simulink model "SIMULACION_DEFINITIVA"  (R2019b)
settings: Solver=VariableStepAuto  StartTime=0.0  StopTime=10.0  RelTol=1e-3
values from neighbouring files (symbols this model uses):
  A = double(A)    [CODIGO_FINAL_PROYECTO.m]
  B = double(B)    [CODIGO_FINAL_PROYECTO.m]
  C = [1 0 0 0;0 0 1 0]    [CODIGO_FINAL_PROYECTO.m]
  K = lqr(A,B,Q,R)    [CODIGO_FINAL_PROYECTO.m]
  L = lqr(A',C',E*Sxi*E',Seta)'    [CODIGO_FINAL_PROYECTO.m]
  r = 0    [CODIGO_FINAL_PROYECTO.m]
  Seta = diag([0.01^2,0.01^2])    [CODIGO_FINAL_PROYECTO.m]
  Sxi = diag([0.05^2,0.05^2])    [CODIGO_FINAL_PROYECTO.m]
  UEQ = 0    [CODIGO_FINAL_PROYECTO.m]
  x0 = [179*pi/180;0;0*pi/180;0]    [CODIGO_FINAL_PROYECTO.m]
  XEQ = [pi;0;0;0]    [CODIGO_FINAL_PROYECTO.m]
  xh0 = [179*pi/180;0;0*pi/180;0]*1.05    [CODIGO_FINAL_PROYECTO.m]
  YEQ = [pi;0]    [CODIGO_FINAL_PROYECTO.m]
settings Model: Creator=Raffa  LastModifiedBy=Raffa

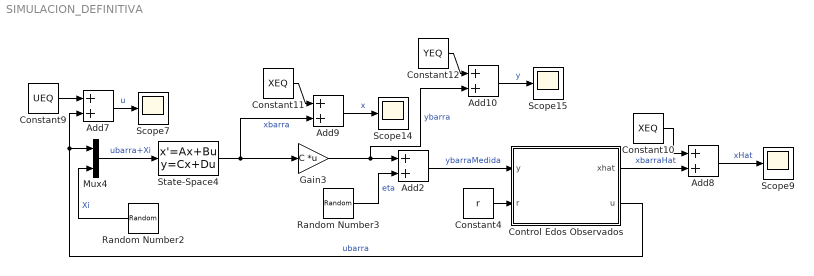
== system SIMULACION_DEFINITIVA ==
  Add{2,7..10} (5 alike) : Sum
  Constant10 : Constant  Value=XEQ
  Constant11 : Constant  Value=XEQ
  Constant12 : Constant  Value=YEQ
  Constant4 : Constant  Value=r  VectorParams1D=off
  Constant9 : Constant  Value=UEQ
  Control Edos Observados : Subsystem
  Gain3 : Gain  Gain=C  Multiplication=Matrix(K*u)
  Mux4 : Mux  Inputs=2
  Random Number2 : RandomNumber  Mean=[0;0]  Variance=[Sxi(1,1);Sxi(2,2)]  Seed=[1;2]  SampleTime=0.001  VectorParams1D=off
  Random Number3 : RandomNumber  Mean=[0;0]  Variance=[Seta(1,1);Seta(2,2)]  Seed=[3;4]  SampleTime=0.001  VectorParams1D=off
  Scope{7,9,14..15} (4 alike) : Scope
  State-Space4 : StateSpace  A=A  B=[B E]  C=eye(4)  D=zeros(4,3)  InitialCondition=x0-XEQ
  wires:
  Control Edos Observados/2(u) -> Add7/2, Mux4/1  "ubarra"
  Mux4/1 -> State-Space4/1  "ubarra+Xi"
  Gain3/1 -> Add10/2, Add2/1  "ybarra"
  Constant10/1 -> Add8/1
  Random Number2/1 -> Mux4/2  "Xi"
  Add8/1 -> Scope9/1  "xHat"
  Add10/1 -> Scope15/1  "y"
  Random Number3/1 -> Add2/2  "eta"
  Add7/1 -> Scope7/1  "u"
  Constant9/1 -> Add7/1
  Add2/1 -> Control Edos Observados/1(y)  "ybarraMedida"
  State-Space4/1 -> Gain3/1, Add9/2  "xbarra"
  Constant11/1 -> Add9/1
  Constant4/1 -> Control Edos Observados/2(r)
  Control Edos Observados/1(xhat) -> Add8/2  "xbarraHat"
  Add9/1 -> Scope14/1  "x"
  Constant12/1 -> Add10/1

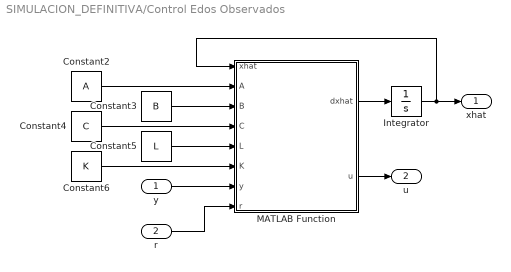
== system SIMULACION_DEFINITIVA/Control Edos Observados ==
  y : Inport
  r : Inport  Port=2
  Constant2 : Constant  Value=A  VectorParams1D=off
  Constant3 : Constant  Value=B  VectorParams1D=off
  Constant4 : Constant  Value=C  VectorParams1D=off
  Constant5 : Constant  Value=L  VectorParams1D=off
  Constant6 : Constant  Value=K  VectorParams1D=off
  Integrator : Integrator  InitialCondition=xh0-XEQ
  MATLAB Function : MATLAB Function  TreatAsAtomicUnit=on
  xhat : Outport
  u : Outport  Port=2
  wires:
  r/1 -> MATLAB Function/8(r)
  y/1 -> MATLAB Function/7(y)
  Constant4/1 -> MATLAB Function/4(C)
  Constant6/1 -> MATLAB Function/6(K)
  Constant5/1 -> MATLAB Function/5(L)
  Integrator/1 -> MATLAB Function/1(xhat), xhat/1
  Constant3/1 -> MATLAB Function/3(B)
  MATLAB Function/1(dxhat) -> Integrator/1
  Constant2/1 -> MATLAB Function/2(A)
  MATLAB Function/2(u) -> u/1

== matlab function SIMULACION_DEFINITIVA/Control Edos Observados/MATLAB Function ==
  data: xhat input; dxhat output; A input; B input; C input; L input; K input; u output; y input; r input
function [dxhat,u] = fcn(xhat,A,B,C,L,K,y,r)

dxhat = (A-L*C-B*K)*xhat + B*r + L*y;
u=-K*xhat+r;

% function xep = fcn(xe,L,u,ym)
% %xe: x estimada
% %ye: y estimada
% %ym: y medida
% Ai=[-2 -6.25;1 4.25];
% B=[0;1]; C=[0 1];
% 
% ye=C*xe; 
% 
% xep = Ai*xe + B*u - L*(ye-ym);
% 
% function [dx,y,yn] = fcn(x,u,xi,eta,A,B,C,E)
% 
% dx=A*x+B*u+E*xi;
% y=C*x;      %Salida sin ruido para simulacion
% yn=y+eta;   %Salida con ruido
